simulink model "IV_2018B_conplex"  (R2018b)
settings: Solver=VariableStepAuto  StartTime=0.0  StopTime=105.0  RelTol=1e-3
libraries: fl_lib x24, nesl_utility x17, elec_lib x2
settings Model: Creator=94840  LastModifiedBy=WangMingcheng
settings DataIOCC: SaveFormat=Array

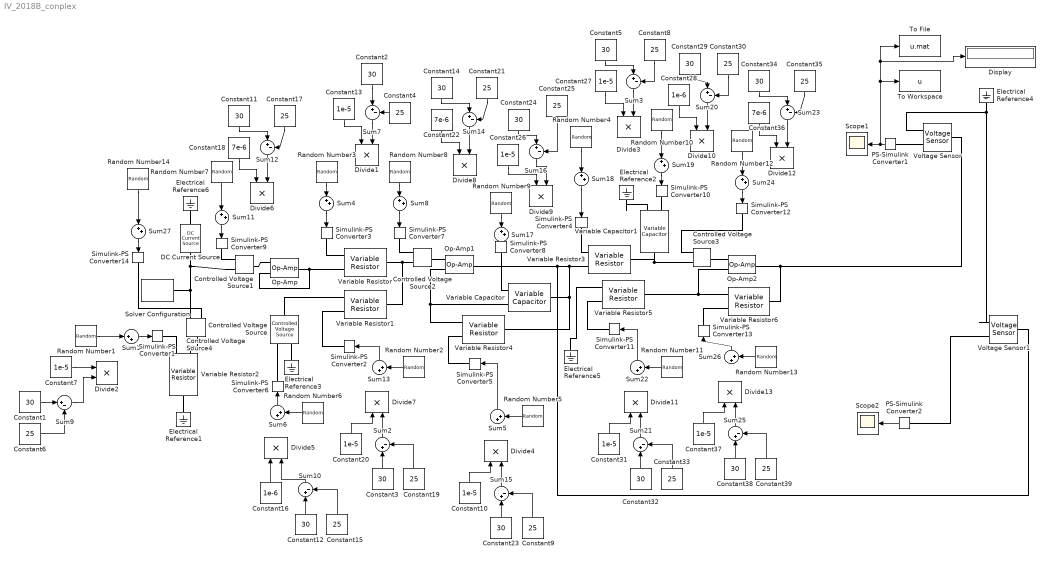
== system IV_2018B_conplex ==
  Constant{1..3,5,11..12,14,23..24,29,32,34,38} (13 alike) : Constant  Value=30
  Constant{7,10,13,20,26..27,31,37} (8 alike) : Constant  Value=1e-5
  Constant{4,6,8..9,15,17,19,21,25,30,33,35,39} (13 alike) : Constant  Value=25
  Constant16 : Constant  Value=1e-6
  Constant18 : Constant  Value=7e-6
  Constant22 : Constant  Value=7e-6
  Constant28 : Constant  Value=1e-6
  Constant36 : Constant  Value=7e-6
  Controlled Voltage Source{,1..4} (5 alike) : fl_lib/Electrical/Electrical Sources/Controlled Voltage Source
  DC Current Source : fl_lib/Electrical/Electrical Sources/DC Current Source  i0=0.15 A
      settings: SourceProductName=Simscape  SourceProductBaseCode=SS
  Display : Display
  Divide{1..13} (13 alike) : Product  Inputs=**
  Electrical Reference{1..6} (6 alike) : fl_lib/Electrical/Electrical Elements/Electrical Reference
  Op-Amp : fl_lib/Electrical/Electrical Elements/Op-Amp  outI_specify=off  outI_priority=None  outI=0 A  outI_nominal_specify=off  outI_nominal_unit=A  outI_nominal_value=1
  Op-Amp1 : fl_lib/Electrical/Electrical Elements/Op-Amp  outI_specify=off  outI_priority=None  outI=0 A  outI_nominal_specify=off  outI_nominal_unit=A  outI_nominal_value=1
  Op-Amp2 : fl_lib/Electrical/Electrical Elements/Op-Amp  outI_specify=off  outI_priority=None  outI=0 A  outI_nominal_specify=off  outI_nominal_unit=A  outI_nominal_value=1
  PS-Simulink Converter1 : nesl_utility/PS-Simulink Converter  PhysicalDomain=network_engine_domain  SubClassName=ps_output  LeftPortType=input  RightPortType=output  PseudoPeriodic=off  Frequencies=[]  Unit=1  AffineConversion=off
  PS-Simulink Converter2 : nesl_utility/PS-Simulink Converter  PhysicalDomain=network_engine_domain  SubClassName=ps_output  LeftPortType=input  RightPortType=output  PseudoPeriodic=off  Frequencies=[]  Unit=1  AffineConversion=off
  Random Number1 : RandomNumber  Mean=10  Variance=0.0  Seed=698  SampleTime=0.001
  Random Number10 : RandomNumber  Mean=5e-5  Variance=0.0  Seed=843  SampleTime=0.001
  Random Number11 : RandomNumber  Mean=1000000  Variance=0.0  Seed=231  SampleTime=0.001
  Random Number12 : RandomNumber  Variance=0.0  Seed=256  SampleTime=0.001
  Random Number13 : RandomNumber  Mean=1  Variance=0.0  Seed=508  SampleTime=0.001
  Random Number14 : RandomNumber  Variance=0  SampleTime=0.001
  Random Number2 : RandomNumber  Mean=10000  Variance=0.0  Seed=711  SampleTime=0.001  VectorParams1D=off
  Random Number3 : RandomNumber  Mean=10000  Variance=0.0  Seed=980  SampleTime=0.001
  Random Number4 : RandomNumber  Mean=10000  Variance=0.0  Seed=395  SampleTime=0.001
  Random Number5 : RandomNumber  Mean=5100  Variance=0.0  Seed=162  SampleTime=0.001
  Random Number6 : RandomNumber  Mean=3.3  Variance=0.0  Seed=853  SampleTime=0.001
  Random Number7 : RandomNumber  Variance=0.0  Seed=320  SampleTime=0.001
  Random Number8 : RandomNumber  Variance=0.0  Seed=909  SampleTime=0.001
  Random Number9 : RandomNumber  Mean=1e-5  Variance=0.0  Seed=579  SampleTime=0.001  VectorParams1D=off
  Scope1 : Scope
  Scope2 : Scope
  Simulink-PS Converter{1..14} (14 alike) : nesl_utility/Simulink-PS Converter  PhysicalDomain=network_engine_domain  SubClassName=ps_input  LeftPortType=input  RightPortType=output  PseudoPeriodic=off  Frequencies=[]  NoiseDistribution=none  NoiseParameters=[]  Unit=1  AffineConversion=off  FilteringAndDerivatives=provide  SimscapeFilterOrder=1  InputFilterTimeConstant=0.001  UdotUserProvided=0
  Solver Configuration : nesl_utility/Solver Configuration  PhysicalDomain=network_engine_domain  SubClassName=solver  LeftPortType=input  RightPortType=generic  Tones=[]  Harmonics=[]  SimulateNoise=off  Profile=off  UseLocalSampling=off  EnableSwitchedLinearOptims=on  FrequencyDomain=off  UseCCode=off  RelTol=0.001  AbsTol=1e-06  MinStep=1e-09  ToWorkspace=off  RevertToSquareIcSolve=off  NumHomotopyIterations=100  PhasorMode=off  PhasorModeNumHarmonics=1  DoDC=on  ResidualTolerance=1e-09  UseLocalSolver=on  LocalSolverChoice=NE_BACKWARD_EULER_ADVANCER  LocalSolverSampleTime=0.001  DoFixedCost=on  MaxNonlinIter=3  MaxModeIter=2  LinearAlgebra=auto  EquationFormulation=NE_TIME_EF  DelaysMemoryBudget=1024  AutomaticFiltering=on  FilteringTimeConstant=0.001  PartitionStorageMethod=AS_NEEDED  PartitionMemoryBudget=1024
  Sum{1,4..6,8,11,13,17..19,22,24,26..27} (14 alike) : Sum  Inputs=|++
  Sum{2..3,7,9..10,12,14..16,20..21,23,25} (13 alike) : Sum  Inputs=|+-
  To File : ToFile  Filename=u.mat
  To Workspace : ToWorkspace  VariableName=u  SampleTime=-1
      settings: MaxDataPoints=100000  Save2DSignal=2-D array (concatenate along first dimension)
  Variable Capacitor : elec_lib/Passive Devices/Variable Capacitor  prm=2  Cmin=0.9 uF  r=1e-6 Ohm  v0=0 V  q0=0 C
      settings: SourceProductName=Simscape Electronics  SourceProductBaseCode=SN
  Variable Capacitor1 : elec_lib/Passive Devices/Variable Capacitor  prm=2  Cmin=45 uF  r=1e-6 Ohm  v0=0 V  q0=0 C
      settings: SourceProductName=Simscape Electronics  SourceProductBaseCode=SN
  Variable Resistor : fl_lib/Electrical/Electrical Elements/Variable Resistor  Rmin=9 kOhm  i_specify=off  i_priority=None  i=0 A  i_nominal_specify=off  i_nominal_unit=A  i_nominal_value=1  v_specify=off  v_priority=None  v=0 V  v_nominal_specify=off  v_nominal_unit=V  v_nominal_value=1
  Variable Resistor1 : fl_lib/Electrical/Electrical Elements/Variable Resistor  Rmin=9 kOhm  i_specify=off  i_priority=None  i=0 A  i_nominal_specify=off  i_nominal_unit=A  i_nominal_value=1  v_specify=off  v_priority=None  v=0 V  v_nominal_specify=off  v_nominal_unit=V  v_nominal_value=1
  Variable Resistor2 : fl_lib/Electrical/Electrical Elements/Variable Resistor  Rmin=9 Ohm  i_specify=off  i_priority=None  i=0 A  i_nominal_specify=off  i_nominal_unit=A  i_nominal_value=1  v_specify=off  v_priority=None  v=0 V  v_nominal_specify=off  v_nominal_unit=V  v_nominal_value=1
  Variable Resistor3 : fl_lib/Electrical/Electrical Elements/Variable Resistor  Rmin=9 kOhm  i_specify=off  i_priority=None  i=0 A  i_nominal_specify=off  i_nominal_unit=A  i_nominal_value=1  v_specify=off  v_priority=None  v=0 V  v_nominal_specify=off  v_nominal_unit=V  v_nominal_value=1
  Variable Resistor4 : fl_lib/Electrical/Electrical Elements/Variable Resistor  Rmin=4.5 kOhm  i_specify=off  i_priority=None  i=0 A  i_nominal_specify=off  i_nominal_unit=A  i_nominal_value=1  v_specify=off  v_priority=None  v=0 V  v_nominal_specify=off  v_nominal_unit=V  v_nominal_value=1
  Variable Resistor5 : fl_lib/Electrical/Electrical Elements/Variable Resistor  Rmin=0.9 MOhm  i_specify=off  i_priority=None  i=0 A  i_nominal_specify=off  i_nominal_unit=A  i_nominal_value=1  v_specify=off  v_priority=None  v=0 V  v_nominal_specify=off  v_nominal_unit=V  v_nominal_value=1
  Variable Resistor6 : fl_lib/Electrical/Electrical Elements/Variable Resistor  Rmin=0.9 Ohm  i_specify=off  i_priority=None  i=0 A  i_nominal_specify=off  i_nominal_unit=A  i_nominal_value=1  v_specify=off  v_priority=None  v=0 V  v_nominal_specify=off  v_nominal_unit=V  v_nominal_value=1
  Voltage Sensor : fl_lib/Electrical/Electrical Sensors/Voltage Sensor
  Voltage Sensor1 : fl_lib/Electrical/Electrical Sensors/Voltage Sensor
  wires:
  Sum1/1 -> Simulink-PS Converter1/1
  PS-Simulink Converter1/1 -> Display/1, To File/1, To Workspace/1, Scope1/1
  Random Number1/1 -> Sum1/1
  Constant7/1 -> Divide2/1
  Sum6/1 -> Simulink-PS Converter6/1
  Random Number6/1 -> Sum6/2
  Constant1/1 -> Sum9/1
  Constant6/1 -> Sum9/2
  Sum9/1 -> Divide2/2
  Constant12/1 -> Sum10/1
  Constant15/1 -> Sum10/2
  Sum10/1 -> Divide5/2
  Constant16/1 -> Divide5/1
  Sum11/1 -> Simulink-PS Converter9/1
  Constant11/1 -> Sum12/1
  Random Number7/1 -> Sum11/1
  Constant17/1 -> Sum12/2
  Sum12/1 -> Divide6/2
  Constant18/1 -> Divide6/1
  Constant2/1 -> Sum7/1
  Random Number3/1 -> Sum4/1
  Sum4/1 -> Simulink-PS Converter3/1
  Sum7/1 -> Divide1/2
  Constant4/1 -> Sum7/2
  Constant13/1 -> Divide1/1
  Random Number2/1 -> Sum13/2
  Constant20/1 -> Divide7/1
  Constant19/1 -> Sum2/2
  Constant3/1 -> Sum2/1
  Sum13/1 -> Simulink-PS Converter2/1
  Constant14/1 -> Sum14/1
  Random Number8/1 -> Sum8/1
  Sum8/1 -> Simulink-PS Converter7/1
  Sum14/1 -> Divide8/2
  Constant21/1 -> Sum14/2
  Constant22/1 -> Divide8/1
  Constant10/1 -> Divide4/1
  Constant23/1 -> Sum15/1
  Constant9/1 -> Sum15/2
  Sum15/1 -> Divide4/2
  Sum5/1 -> Simulink-PS Converter5/1
  Random Number5/1 -> Sum5/2
  Random Number9/1 -> Sum17/1
  Sum17/1 -> Simulink-PS Converter8/1
  Constant24/1 -> Sum16/1
  Constant26/1 -> Divide9/1
  Constant25/1 -> Sum16/2
  Sum16/1 -> Divide9/2
  Sum3/1 -> Divide3/2
  Constant8/1 -> Sum3/2
  Constant5/1 -> Sum3/1
  Constant27/1 -> Divide3/1
  Random Number4/1 -> Sum18/1
  Sum18/1 -> Simulink-PS Converter4/1
  Constant29/1 -> Sum20/1
  Constant30/1 -> Sum20/2
  Sum20/1 -> Divide10/2
  Random Number10/1 -> Sum19/1
  Constant28/1 -> Divide10/1
  Sum19/1 -> Simulink-PS Converter10/1
  Constant31/1 -> Divide11/1
  Constant32/1 -> Sum21/1
  Constant33/1 -> Sum21/2
  Sum22/1 -> Simulink-PS Converter11/1
  Sum21/1 -> Divide11/2
  Random Number11/1 -> Sum22/2
  Random Number12/1 -> Sum24/1
  Sum24/1 -> Simulink-PS Converter12/1
  Constant34/1 -> Sum23/1
  Constant36/1 -> Divide12/1
  Constant35/1 -> Sum23/2
  Sum23/1 -> Divide12/2
  Random Number13/1 -> Sum26/2
  Constant37/1 -> Divide13/1
  Constant39/1 -> Sum25/2
  Sum25/1 -> Divide13/2
  Constant38/1 -> Sum25/1
  Sum26/1 -> Simulink-PS Converter13/1
  PS-Simulink Converter2/1 -> Scope2/1
  Sum27/1 -> Simulink-PS Converter14/1
  Random Number14/1 -> Sum27/1
  Sum2/1 -> Divide7/2
  connections:
  Controlled Voltage Source1/RConn2 -- DC Current Source/LConn1 -- Controlled Voltage Source4/RConn2 -- Solver Configuration/RConn1
  Simulink-PS Converter1/RConn1 -- Variable Resistor2/LConn1
  Simulink-PS Converter2/RConn1 -- Variable Resistor1/LConn1
  Electrical Reference1/LConn1 -- Variable Resistor2/RConn1
  Variable Resistor1/LConn2 -- Controlled Voltage Source/LConn1
  Electrical Reference3/LConn1 -- Controlled Voltage Source/RConn2
  Variable Resistor/RConn1 -- Variable Resistor1/RConn1 -- Controlled Voltage Source2/RConn2
  Variable Resistor3/LConn2 -- Voltage Sensor1/LConn1 -- Op-Amp1/RConn1 -- Variable Resistor4/RConn1 -- Variable Capacitor/RConn1
  Voltage Sensor/RConn2 -- Voltage Sensor1/RConn2 -- Electrical Reference4/LConn1
  PS-Simulink Converter1/LConn1 -- Voltage Sensor/RConn1
  Simulink-PS Converter4/RConn1 -- Variable Resistor3/LConn1
  Simulink-PS Converter5/RConn1 -- Variable Resistor4/LConn1
  Electrical Reference6/LConn1 -- DC Current Source/RConn1
  Op-Amp/RConn1 -- Variable Resistor/LConn2 -- Op-Amp/LConn2
  Simulink-PS Converter6/RConn1 -- Controlled Voltage Source/RConn1
  Variable Resistor4/LConn2 -- Op-Amp1/LConn2 -- Variable Capacitor/LConn2
  Op-Amp/LConn1 -- Controlled Voltage Source1/LConn1
  Simulink-PS Converter3/RConn1 -- Variable Resistor/LConn1
  Op-Amp1/LConn1 -- Controlled Voltage Source2/LConn1
  Simulink-PS Converter8/RConn1 -- Variable Capacitor/LConn1
  Variable Capacitor1/RConn1 -- Variable Resistor3/RConn1 -- Controlled Voltage Source3/RConn2
  Simulink-PS Converter10/RConn1 -- Variable Capacitor1/LConn1
  Electrical Reference2/LConn1 -- Variable Capacitor1/LConn2
  Simulink-PS Converter11/RConn1 -- Variable Resistor5/LConn1
  Variable Resistor5/RConn1 -- Variable Resistor6/LConn2 -- Op-Amp2/LConn2
  Electrical Reference5/LConn1 -- Variable Resistor5/LConn2
  Variable Resistor6/RConn1 -- Op-Amp2/RConn1 -- Voltage Sensor/LConn1
  Controlled Voltage Source3/LConn1 -- Op-Amp2/LConn1
  Simulink-PS Converter13/RConn1 -- Variable Resistor6/LConn1
  PS-Simulink Converter2/LConn1 -- Voltage Sensor1/RConn1
  Controlled Voltage Source4/LConn1 -- Variable Resistor2/LConn2
  Simulink-PS Converter7/RConn1 -- Controlled Voltage Source2/RConn1
  Simulink-PS Converter9/RConn1 -- Controlled Voltage Source1/RConn1
  Controlled Voltage Source4/RConn1 -- Simulink-PS Converter14/RConn1
  Simulink-PS Converter12/RConn1 -- Controlled Voltage Source3/RConn1
